simulink model "sugen"  (R2022b)
settings: Solver=FixedStepAuto  StartTime=0.0  StopTime=600  FixedStep=1  RelTol=1e-3
values from neighbouring files (symbols this model uses):
  Kd_kapa = Kp*Td/Ku_kapa    (= 10.9347)    [Parametri.m]
  Kp = 0.6*Kkr    (= 73.8)    [Parametri.m]
  Kp_kapa = Kp/Ku_kapa    (= 9.84)    [Parametri.m]
  Kp_kapa_1 = Kp/Ku_kapa_1    (= 4.92)    [Parametri.m]
  Ku_kapa = 7.5    [Parametri.m]
  Ku_kapa_1 = 15    [Parametri.m]
  Td = Tkr/8    (= 1.11125)    [Parametri.m]
  Ti = Tkr/2    (= 4.445)    [Parametri.m]
libraries: fuzblock x2
settings Model: Creator=Dragana  LastModifiedBy=nd190052d
settings DebuggingCC: UnconnectedInputMsg=warning  UnconnectedOutputMsg=warning  UnconnectedLineMsg=warning
settings ModelReferenceCC: EnableRefExpFcnMdlSchedulingChecks=on
settings RTWCC: DLArmComputeVersion=19.05

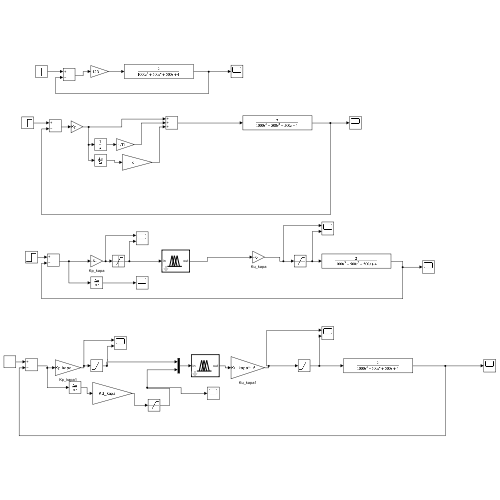
[thumbnail: Simulink's stored preview of the top-level diagram]
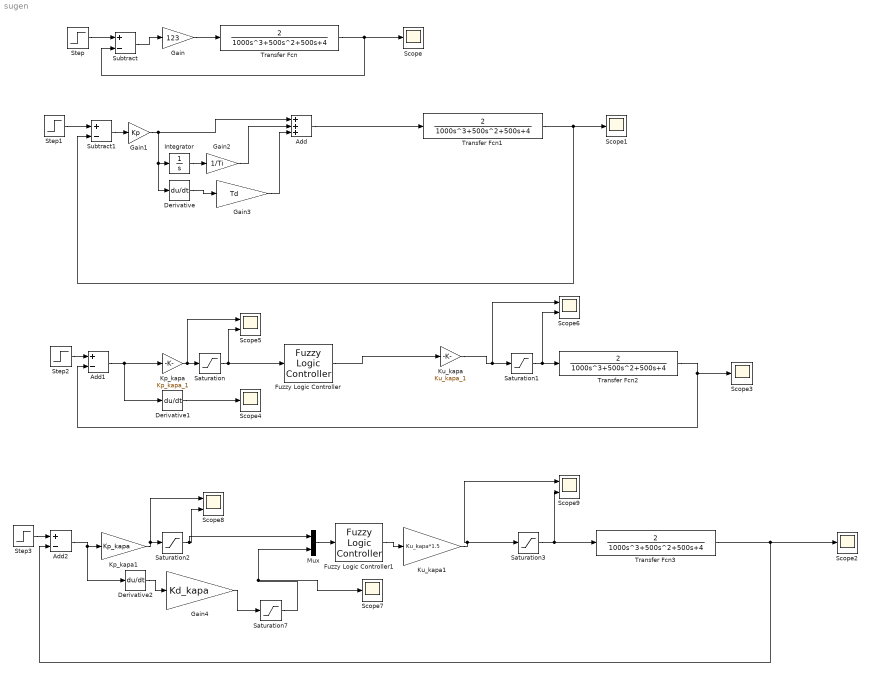
== system sugen ==
  Add : Sum  Inputs=+++
  Add1 : Sum  Inputs=+-
  Add2 : Sum  Inputs=+-
  Derivative : Derivative
  Derivative1 : Derivative
  Derivative2 : Derivative
  Fuzzy Logic Controller : fuzblock/Fuzzy Logic  Controller  FIS='sugenoP.fis'  OutputSampleNumber=101  DataType=double  FuzzifiedInputs=off  RuleFiringStrengths=off  RuleOutputs=off  AggregatedOutputs=off  SimulateUsing=Interpreted execution  OutOfRangeInputValueMessage=warning  NoRuleFiredMessage=warning  EmptyOutputFuzzySetMessage=warning
  Fuzzy Logic Controller1 : fuzblock/Fuzzy Logic  Controller  FIS='sugenoPIDnelin.fis'  OutputSampleNumber=101  DataType=double  FuzzifiedInputs=off  RuleFiringStrengths=off  RuleOutputs=off  AggregatedOutputs=off  SimulateUsing=Interpreted execution  OutOfRangeInputValueMessage=warning  NoRuleFiredMessage=warning  EmptyOutputFuzzySetMessage=warning
  Gain : Gain  Gain=123
  Gain1 : Gain  Gain=Kp
  Gain2 : Gain  Gain=1/Ti
  Gain3 : Gain  Gain=Td
  Gain4 : Gain  Gain=Kd_kapa
  Integrator : Integrator
  Kp_kapa : Gain  Gain=Kp_kapa_1
  Kp_kapa1 : Gain  Gain=Kp_kapa
  Ku_kapa : Gain  Gain=Ku_kapa_1
  Ku_kapa1 : Gain  Gain=Ku_kapa*1.5
  Mux : Mux  Inputs=2
  Saturation{,1..2,7} (4 alike) : Saturate  UpperLimit=1  LowerLimit=-1
  Saturation3 : Saturate  UpperLimit=15  LowerLimit=-15
  Scope{,1..4,7} (6 alike) : Scope
  Scope{5..6,8..9} (4 alike) : Scope  NumInputPorts=2
  Step{,1..3} (4 alike) : Step  Time=200  Before=-3  After=3  SampleTime=0
  Subtract : Sum  Inputs=+-
  Subtract1 : Sum  Inputs=+-
  Transfer Fcn{,1..3} (4 alike) : TransferFcn  Numerator=[2]  Denominator=[1000 500 500 4]
  wires:
  Gain/1 -> Transfer Fcn/1
  Transfer Fcn/1 -> Subtract/2, Scope/1
  Step/1 -> Subtract/1
  Subtract/1 -> Gain/1
  Subtract1/1 -> Gain1/1
  Step1/1 -> Subtract1/1
  Transfer Fcn1/1 -> Subtract1/2, Scope1/1
  Gain1/1 -> Derivative/1, Integrator/1, Add/1
  Add/1 -> Transfer Fcn1/1
  Derivative/1 -> Gain3/1
  Integrator/1 -> Gain2/1
  Gain2/1 -> Add/2
  Gain3/1 -> Add/3
  Step2/1 -> Add1/1
  Add1/1 -> Derivative1/1, Kp_kapa/1
  Kp_kapa/1 -> Scope5/1, Saturation/1
  Ku_kapa/1 -> Scope6/1, Saturation1/1
  Fuzzy Logic Controller/1 -> Ku_kapa/1
  Saturation1/1 -> Transfer Fcn2/1, Scope6/2
  Transfer Fcn2/1 -> Scope3/1, Add1/2
  Saturation/1 -> Scope5/2, Fuzzy Logic Controller/1
  Derivative1/1 -> Scope4/1
  Kp_kapa1/1 -> Scope8/1, Saturation2/1
  Add2/1 -> Derivative2/1, Kp_kapa1/1
  Ku_kapa1/1 -> Scope9/1, Saturation3/1
  Saturation3/1 -> Transfer Fcn3/1, Scope9/2
  Derivative2/1 -> Gain4/1
  Fuzzy Logic Controller1/1 -> Ku_kapa1/1
  Transfer Fcn3/1 -> Add2/2, Scope2/1
  Step3/1 -> Add2/1
  Saturation2/1 -> Mux/1, Scope8/2
  Mux/1 -> Fuzzy Logic Controller1/1
  Gain4/1 -> Saturation7/1
  Saturation7/1 -> Mux/2, Scope7/1
